simulink model "Hinf_Sem_Incertezas_Realimentacao_an"  (R2013b)
settings: Solver=ode45  StartTime=0.0  StopTime=10.0  RelTol=1e-3
values from neighbouring files (symbols this model uses):
  An = [-1.02   0.905 ... (first row only)    [Main.m]    (also in Teste_paper_Robusto_ITA_My_Analisis.m)
  Bn = [ -0.0215 ... (first row only)    [Main.m]    (also in Teste_paper_Robusto_ITA_My_Analisis.m)
  Cn = [    0  57.295 ... (first row only)    [Main.m]    (also in Teste_paper_Robusto_ITA_My_Analisis.m)
  den_Hinf = K_tf.den{1}    [Teste_paper_Robusto_ITA_My_Analisis.m]
  Dn = [     0 ... (first row only)    [Main.m]    (also in Teste_paper_Robusto_ITA_My_Analisis.m)
  num_Hinf = K_tf.num{1}    [Teste_paper_Robusto_ITA_My_Analisis.m]
settings Model: Creator=Eduardo  LastModifiedBy=Eduardo

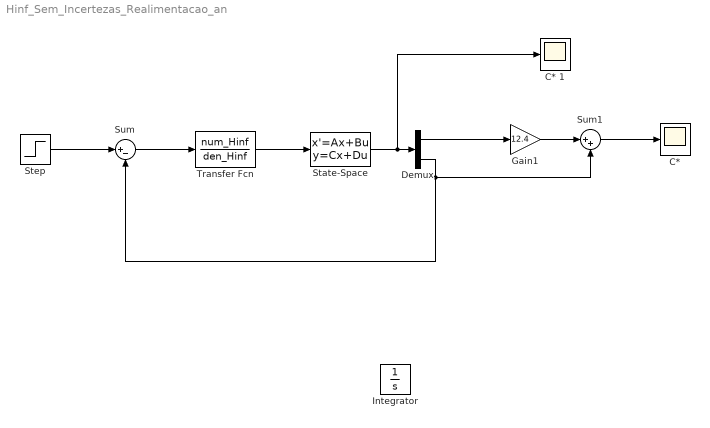
== system Hinf_Sem_Incertezas_Realimentacao_an ==
  "C* " : Scope
  C* 1 : Scope
  Demux : Demux  Outputs=2
  Gain1 : Gain  Gain=12.4
  Integrator : Integrator
  State-Space : StateSpace  A=An  B=Bn  C=Cn  D=Dn  X0=0
  Step : Step  SampleTime=0
  Sum : Sum  Inputs=|+-
  Sum1 : Sum  Inputs=|++
  Transfer Fcn : TransferFcn  Numerator=num_Hinf  Denominator=den_Hinf
  wires:
  State-Space/1 -> C* 1/1, Demux/1
  Step/1 -> Sum/1
  Demux/2 -> Sum1/2, Sum/2
  Sum/1 -> Transfer Fcn/1
  Transfer Fcn/1 -> State-Space/1
  Demux/1 -> Gain1/1
  Gain1/1 -> Sum1/1
  Sum1/1 -> "C* "/1
